simulink model "QP_FXP_2016a"  (R2016a)
settings: Solver=FixedStepAuto  SolverMode=SingleTasking  StartTime=0.0  StopTime=200  FixedStep=0.001  RelTol=1e-3
values from neighbouring files (symbols this model uses):
  KK = lqr(A,B,Q,R)    [Para.m]
libraries: simulink x1
settings Model: Creator=chengqian  LastModifiedBy=chengqian
settings DebuggingCC: SFUnexpectedBacktrackingDiag=error  SFNoUnconditionalDefaultTransitionDiag=error
settings SFSimCC: SimUseLocalCustomCode=on
settings RTWCC: RTWUseLocalCustomCode=on
settings GRTTargetCC: TargetLangStandard=C99 (ISO)  GeneratePreprocessorConditionals=Use local settings
settings ConfigComp: CovMetricSettings=dwe  CovHtmlReporting=off  CovSaveCumulativeToWorkspaceVar=off  CovSaveSingleToWorkspaceVar=off  CovExternalEMLEnable=on

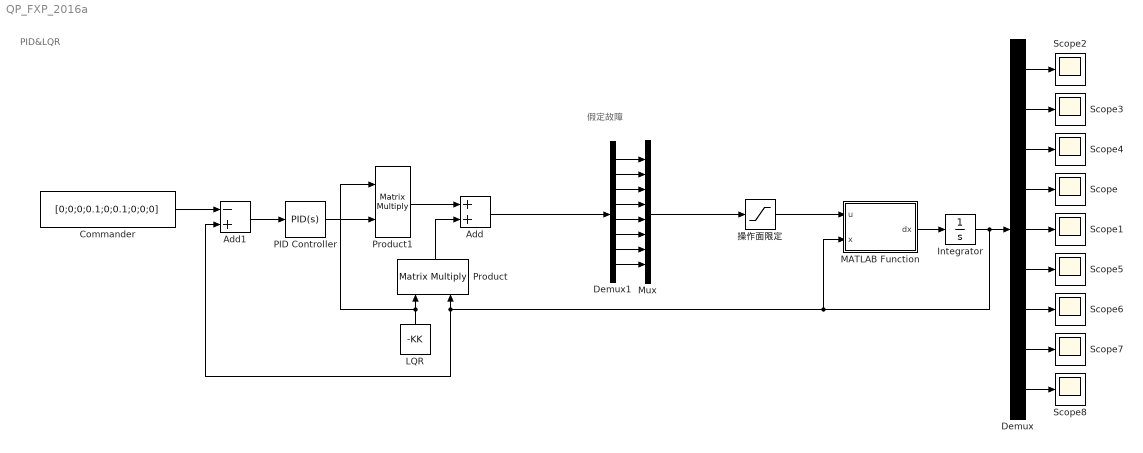
== system QP_FXP_2016a ==
  note: 假定故障
  note: PID&LQR
  Add : Sum
  Add1 : Sum  Inputs=-+
  Commander : Constant  Value=[0;0;0;0.1;0;0.1;0;0;0]
  Demux : Demux  Outputs=9
  Demux1 : Demux  Outputs=8
  Integrator : Integrator  InitialCondition=[0;0;0;0;0;0;0;0;0]
  LQR : Constant  Value=-KK
  MATLAB Function : MATLAB Function  TreatAsAtomicUnit=on
  Mux : Mux  Inputs=8
  PID Controller : simulink/Continuous/PID Controller  Controller=PID  Form=Parallel  TimeDomain=Continuous-time  SampleTime=-1  IntegratorMethod=Forward Euler  FilterMethod=Forward Euler  ControllerParametersSource=internal  P=[0;0;0;30;0;0;0;0;0]  I=[0;0;2;16;0;0;0;0;0]  D=[0;0;0;5;0;0;0;0;0]  UseFilter=on  N=1000  InitialConditionSource=internal  InitialConditionForIntegrator=0  InitialConditionForFilter=0  DifferentiatorICPrevScaledInput=0  ExternalReset=none  TrackingMode=off  Kt=1  LimitOutput=off  UpperSaturationLimit=inf  LowerSaturationLimit=-inf  LinearizeAsGain=on  AntiWindupMode=none  Kb=1  POutMin=[]  POutMax=[]  IOutMin=[]  IOutMax=[]  DOutMin=[]  DOutMax=[]  NOutMin=[]  NOutMax=[]  SumOutMin=[]  SumOutMax=[]  SaturationOutMin=[]  SaturationOutMax=[]  PParamMin=[]  PParamMax=[]  IParamMin=[]  IParamMax=[]  DParamMin=[]  DParamMax=[]  NParamMin=[]  NParamMax=[]  KbParamMin=[]  KbParamMax=[]  KtParamMin=[]  KtParamMax=[]  KbOutMin=[]  KbOutMax=[]  KtOutMin=[]  KtOutMax=[]  IntegratorOutMin=[]  IntegratorOutMax=[]  FilterOutMin=[]  FilterOutMax=[]  SumI1OutMin=[]  SumI1OutMax=[]  SumI2OutMin=[]  SumI2OutMax=[]  SumI3OutMin=[]  SumI3OutMax=[]  SumDOutMin=[]  SumDOutMax=[]  DifferentiatorOutMin=[]  DifferentiatorOutMax=[]  IntegratorContinuousStateAttributes=''  IntegratorStateMustResolveToSignalObject=off  IntegratorRTWStateStorageClass=Auto  FilterContinuousStateAttributes=''  FilterStateMustResolveToSignalObject=off  FilterRTWStateStorageClass=Auto
  Product : Product  Multiplication=Matrix(*)
  Product1 : Product  Multiplication=Matrix(*)
  Scope{,1..8} (9 alike) : Scope
  操作面限定 : Saturate  UpperLimit=[25;25;26;26;30;30;30;30]  LowerLimit=-[25;25;15;15;60;60;30;30]
  wires:
  MATLAB Function/1(dx) -> Integrator/1
  LQR/1 -> Product1/1, Product/1
  Integrator/1 -> Demux/1, MATLAB Function/2(x), Add1/2, Product/2
  Product/1 -> Add/2
  PID Controller/1 -> Product1/2
  Add1/1 -> PID Controller/1
  Commander/1 -> Add1/1
  Demux/4 -> Scope/1
  Product1/1 -> Add/1
  Add/1 -> Demux1/1
  Demux/5 -> Scope1/1
  Demux1/1 -> Mux/1
  Demux1/2 -> Mux/2
  Demux1/3 -> Mux/3
  Demux1/5 -> Mux/5
  Demux1/6 -> Mux/6
  Demux1/7 -> Mux/7
  Mux/1 -> 操作面限定/1
  Demux1/8 -> Mux/8
  操作面限定/1 -> MATLAB Function/1(u)
  Demux1/4 -> Mux/4
  Demux/1 -> Scope2/1
  Demux/2 -> Scope3/1
  Demux/3 -> Scope4/1
  Demux/6 -> Scope5/1
  Demux/9 -> Scope8/1
  Demux/8 -> Scope7/1
  Demux/7 -> Scope6/1

== matlab function QP_FXP_2016a/MATLAB Function ==
  data: u input size=8; dx output size=9; x input
function dx = fcn(u,x)

%%x = [p;r;beta;phi;psi;alpha;q;theta;v].
%%u = [delta_rei;delta_lei;delta_rfl;delta_lfl;delta_rvr;delta_lvr;delta_reo;delta_leo]

Alat = [-0.099170  0.020570  2.805001  0.000001 0.000001;
        -0.002640 -0.031920 -0.674200  0        0;
        -0.108500 -0.994000 -0.029750  0.010210 0.000034;
         1.0       0.016090 -0.000148  0.000016 0;
         0         1.0       0.000120 -0.000013 0.000122];
Alon = [-0.064190   1.000001 0.000844 -0.000130;
        -1.424000  -0.051730 0.000001  0;
        -0.0000138  1.0      0.000014  0.000003;
        -0.550041   0       -0.559090 -0.013375];

A = [Alat zeros(5,4);
     zeros(4,5) Alon];
B = [-0.2883  0.2883 -0.8654  0.8654 -0.0000  0.0025 -0.2883  0.2883;
     -0.0959  0.0959  0.2079 -0.2079 -0.0045 -0.0051 -0.0959  0.0959;
      0.0000  0.0000  0.0003 -0.0003 -0.0001  0       0       0;
      0       0       0       0       0       0       0       0;
      0       0       0       0       0       0       0       0;
     -0.0005 -0.0005 -0.0019 -0.0019 -0.0005  0.0004 -0.0005 -0.0005;
     -0.0857 -0.0857 -0.5263 -0.5263  0.0098 -0.0073 -0.0857 -0.0857;
      0       0       0       0       0       0       0       0;
     -0.0034 -0.0034 -0.1285 -0.1285  0.0011 -0.0011 -0.0041 -0.0041]; 

dx = A*x + B*u;
